simulink model "IFACS_Spring2026"  (R2025b)
settings: Solver=ode23t  StartTime=0.0  StopTime=3600*24*3  FixedStep=1  RelTol=1e-3  AbsTol=1e-3
values from neighbouring files (symbols this model uses):
  ac_cooling_capacity = 5000    [IFACS_Constants.m]
  ac_power = ac_cooling_capacity / ac_COP    (= 1250)    [IFACS_Constants.m]
  house_H = 6    [IFACS_Constants.m]
  house_L = 20    [IFACS_Constants.m]
  house_W = 10    [IFACS_Constants.m]
  roof_pitch = 15    [IFACS_Constants.m]
  TinIC = 24    [IFACS_Constants.m]
libraries: fl_lib x215, nesl_utility x52, simulink_extras x29, SimscapeFluids_lib x3
(part 4 of 5)

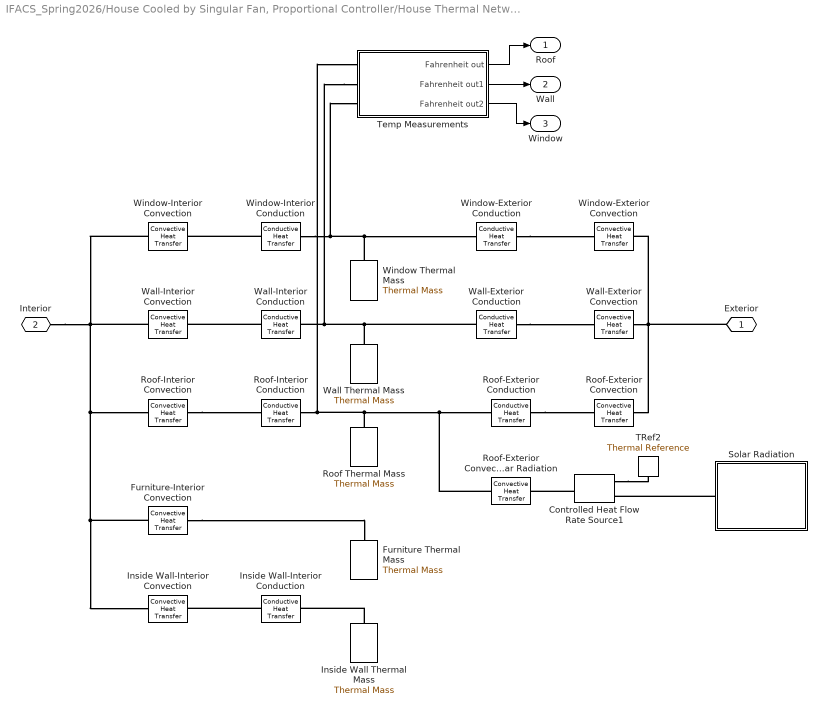
== system IFACS_Spring2026/House Cooled by Singular Fan, Proportional Controller/House Thermal Network/House Thermal Network ==
  Controlled Heat Flow Rate Source1 : fl_lib/Thermal/Thermal Sources/Controlled Heat Flow Rate Source
  Furniture Thermal Mass : fl_lib/Thermal/Thermal Elements/Thermal Mass  mass_type=foundation.enum.constant_variable.constant  mass=M_furniture kg  sp_heat=cp_furniture J/(K*kg)  mass_min=1e-6 kg  num_ports=foundation.enum.numPorts2.one  m_specify=off  m_priority=High  m=1 kg  m_nominal_specify=off  m_nominal_value=1  m_nominal_unit=kg  T_specify=on  T_priority=High  T=T_init_furniture degC  T_nominal_specify=off  T_nominal_value=1  T_nominal_unit=K  Q_specify=off  Q_priority=None  Q=0 W  Q_nominal_specify=off  Q_nominal_value=1  Q_nominal_unit=W
  Furniture-Interior Convection : fl_lib/Thermal/Thermal Elements/Convective Heat Transfer  thermal_type=foundation.enum.constant_variable.constant  area=area_furniture m^2  heat_tr_coeff=hc_furniture_interior W/(K*m^2)  min_heat_tr_coeff=1e-3 W/(K*m^2)  T_specify=off  T_priority=None  T=0 K  T_nominal_specify=off  T_nominal_value=1  T_nominal_unit=K  Q_specify=off  Q_priority=None  Q=0 W  Q_nominal_specify=off  Q_nominal_value=1  Q_nominal_unit=W
  Inside Wall Thermal Mass : fl_lib/Thermal/Thermal Elements/Thermal Mass  mass_type=foundation.enum.constant_variable.constant  mass=rho_wall_inside * area_wall_inside * thickness_wall_inside kg  sp_heat=cp_wall_inside J/(K*kg)  mass_min=1e-6 kg  num_ports=foundation.enum.numPorts2.one  m_specify=off  m_priority=High  m=1 kg  m_nominal_specify=off  m_nominal_value=1  m_nominal_unit=kg  T_specify=on  T_priority=High  T=T_init_wall_inside degC  T_nominal_specify=off  T_nominal_value=1  T_nominal_unit=K  Q_specify=off  Q_priority=None  Q=0 W  Q_nominal_specify=off  Q_nominal_value=1  Q_nominal_unit=W
  Inside Wall-Interior Conduction : fl_lib/Thermal/Thermal Elements/Conductive Heat Transfer  thermal_type=foundation.enum.ConstantVariableTabulated.Constant  wall_geometry=foundation.enum.ConductionWallGeometry.Planar  area=2 * area_wall_inside m^2  thickness=thickness_wall_inside / 2 m  d_in=0.05 m  d_out=0.1 m  L=1 m  th_cond_min=10 W/(K*m)  th_cond=k_wall_inside W/(K*m)  th_cond_TLU=[413, 401, 392, 383, 371, 357, 342] W/(K*m)  temp_TLU=[200, 273, 400, 600, 800, 1000, 1200] K  T_specify=off  T_priority=None  T=0 K  T_nominal_specify=off  T_nominal_value=1  T_nominal_unit=K  Q_specify=off  Q_priority=None  Q=0 W  Q_nominal_specify=off  Q_nominal_value=1  Q_nominal_unit=W
  Inside Wall-Interior Convection : fl_lib/Thermal/Thermal Elements/Convective Heat Transfer  thermal_type=foundation.enum.constant_variable.constant  area=2 * area_wall_inside m^2  heat_tr_coeff=hc_wall_inside_interior W/(K*m^2)  min_heat_tr_coeff=1e-3 W/(K*m^2)  T_specify=off  T_priority=None  T=0 K  T_nominal_specify=off  T_nominal_value=1  T_nominal_unit=K  Q_specify=off  Q_priority=None  Q=0 W  Q_nominal_specify=off  Q_nominal_value=1  Q_nominal_unit=W
  Roof Thermal Mass : fl_lib/Thermal/Thermal Elements/Thermal Mass  mass_type=foundation.enum.constant_variable.constant  mass=rho_roof * area_roof * thickness_roof kg  sp_heat=cp_roof J/(K*kg)  mass_min=1e-6 kg  num_ports=foundation.enum.numPorts2.one  m_specify=off  m_priority=High  m=1 kg  m_nominal_specify=off  m_nominal_value=1  m_nominal_unit=kg  T_specify=on  T_priority=High  T=T_init_roof degC  T_nominal_specify=off  T_nominal_value=1  T_nominal_unit=K  Q_specify=off  Q_priority=None  Q=0 W  Q_nominal_specify=off  Q_nominal_value=1  Q_nominal_unit=W
  Roof-Exterior Conduction : fl_lib/Thermal/Thermal Elements/Conductive Heat Transfer  thermal_type=foundation.enum.ConstantVariableTabulated.Constant  wall_geometry=foundation.enum.ConductionWallGeometry.Planar  area=area_roof m^2  thickness=thickness_roof / 2 m  d_in=0.05 m  d_out=0.1 m  L=1 m  th_cond_min=10 W/(K*m)  th_cond=k_roof W/(K*m)  th_cond_TLU=[413, 401, 392, 383, 371, 357, 342] W/(K*m)  temp_TLU=[200, 273, 400, 600, 800, 1000, 1200] K  T_specify=off  T_priority=None  T=0 K  T_nominal_specify=off  T_nominal_value=1  T_nominal_unit=K  Q_specify=off  Q_priority=None  Q=0 W  Q_nominal_specify=off  Q_nominal_value=1  Q_nominal_unit=W
  Roof-Exterior Convection : fl_lib/Thermal/Thermal Elements/Convective Heat Transfer  thermal_type=foundation.enum.constant_variable.constant  area=area_roof m^2  heat_tr_coeff=hc_roof_exterior W/(K*m^2)  min_heat_tr_coeff=1e-3 W/(K*m^2)  T_specify=off  T_priority=None  T=0 K  T_nominal_specify=off  T_nominal_value=1  T_nominal_unit=K  Q_specify=off  Q_priority=None  Q=0 W  Q_nominal_specify=off  Q_nominal_value=1  Q_nominal_unit=W
  Roof-Exterior Convection Solar Radiation : fl_lib/Thermal/Thermal Elements/Convective Heat Transfer  thermal_type=foundation.enum.constant_variable.constant  area=area_roof m^2  heat_tr_coeff=1 W/(K*m^2)  min_heat_tr_coeff=1e-3 W/(K*m^2)  T_specify=off  T_priority=None  T=0 K  T_nominal_specify=off  T_nominal_value=1  T_nominal_unit=K  Q_specify=off  Q_priority=None  Q=0 W  Q_nominal_specify=off  Q_nominal_value=1  Q_nominal_unit=W
  Roof-Interior Conduction : fl_lib/Thermal/Thermal Elements/Conductive Heat Transfer  thermal_type=foundation.enum.ConstantVariableTabulated.Constant  wall_geometry=foundation.enum.ConductionWallGeometry.Planar  area=area_roof m^2  thickness=thickness_roof / 2 m  d_in=0.05 m  d_out=0.1 m  L=1 m  th_cond_min=10 W/(K*m)  th_cond=k_roof W/(K*m)  th_cond_TLU=[413, 401, 392, 383, 371, 357, 342] W/(K*m)  temp_TLU=[200, 273, 400, 600, 800, 1000, 1200] K  T_specify=off  T_priority=None  T=0 K  T_nominal_specify=off  T_nominal_value=1  T_nominal_unit=K  Q_specify=off  Q_priority=None  Q=0 W  Q_nominal_specify=off  Q_nominal_value=1  Q_nominal_unit=W
  Roof-Interior Convection : fl_lib/Thermal/Thermal Elements/Convective Heat Transfer  thermal_type=foundation.enum.constant_variable.constant  area=area_roof m^2  heat_tr_coeff=hc_roof_interior W/(K*m^2)  min_heat_tr_coeff=1e-3 W/(K*m^2)  T_specify=off  T_priority=None  T=0 K  T_nominal_specify=off  T_nominal_value=1  T_nominal_unit=K  Q_specify=off  Q_priority=None  Q=0 W  Q_nominal_specify=off  Q_nominal_value=1  Q_nominal_unit=W
  Solar Radiation : Subsystem
  TRef2 : fl_lib/Thermal/Thermal Elements/Thermal Reference
  Temp Measurements : Subsystem
  Wall Thermal Mass : fl_lib/Thermal/Thermal Elements/Thermal Mass  mass_type=foundation.enum.constant_variable.constant  mass=rho_wall * area_wall * thickness_wall kg  sp_heat=cp_wall J/(K*kg)  mass_min=1e-6 kg  num_ports=foundation.enum.numPorts2.one  m_specify=off  m_priority=High  m=1 kg  m_nominal_specify=off  m_nominal_value=1  m_nominal_unit=kg  T_specify=on  T_priority=High  T=T_init_wall degC  T_nominal_specify=off  T_nominal_value=1  T_nominal_unit=K  Q_specify=off  Q_priority=None  Q=0 W  Q_nominal_specify=off  Q_nominal_value=1  Q_nominal_unit=W
  Wall-Exterior Conduction : fl_lib/Thermal/Thermal Elements/Conductive Heat Transfer  thermal_type=foundation.enum.ConstantVariableTabulated.Constant  wall_geometry=foundation.enum.ConductionWallGeometry.Planar  area=area_wall m^2  thickness=thickness_wall / 2 m  d_in=0.05 m  d_out=0.1 m  L=1 m  th_cond_min=10 W/(K*m)  th_cond=k_wall W/(K*m)  th_cond_TLU=[413, 401, 392, 383, 371, 357, 342] W/(K*m)  temp_TLU=[200, 273, 400, 600, 800, 1000, 1200] K  T_specify=off  T_priority=None  T=0 K  T_nominal_specify=off  T_nominal_value=1  T_nominal_unit=K  Q_specify=off  Q_priority=None  Q=0 W  Q_nominal_specify=off  Q_nominal_value=1  Q_nominal_unit=W
  Wall-Exterior Convection : fl_lib/Thermal/Thermal Elements/Convective Heat Transfer  thermal_type=foundation.enum.constant_variable.constant  area=area_wall m^2  heat_tr_coeff=hc_wall_exterior W/(K*m^2)  min_heat_tr_coeff=1e-3 W/(K*m^2)  T_specify=off  T_priority=None  T=0 K  T_nominal_specify=off  T_nominal_value=1  T_nominal_unit=K  Q_specify=off  Q_priority=None  Q=0 W  Q_nominal_specify=off  Q_nominal_value=1  Q_nominal_unit=W
  Wall-Interior Conduction : fl_lib/Thermal/Thermal Elements/Conductive Heat Transfer  thermal_type=foundation.enum.ConstantVariableTabulated.Constant  wall_geometry=foundation.enum.ConductionWallGeometry.Planar  area=area_wall m^2  thickness=thickness_wall / 2 m  d_in=0.05 m  d_out=0.1 m  L=1 m  th_cond_min=10 W/(K*m)  th_cond=k_wall W/(K*m)  th_cond_TLU=[413, 401, 392, 383, 371, 357, 342] W/(K*m)  temp_TLU=[200, 273, 400, 600, 800, 1000, 1200] K  T_specify=off  T_priority=None  T=0 K  T_nominal_specify=off  T_nominal_value=1  T_nominal_unit=K  Q_specify=off  Q_priority=None  Q=0 W  Q_nominal_specify=off  Q_nominal_value=1  Q_nominal_unit=W
  Wall-Interior Convection : fl_lib/Thermal/Thermal Elements/Convective Heat Transfer  thermal_type=foundation.enum.constant_variable.constant  area=area_wall m^2  heat_tr_coeff=hc_wall_interior W/(K*m^2)  min_heat_tr_coeff=1e-3 W/(K*m^2)  T_specify=off  T_priority=None  T=0 K  T_nominal_specify=off  T_nominal_value=1  T_nominal_unit=K  Q_specify=off  Q_priority=None  Q=0 W  Q_nominal_specify=off  Q_nominal_value=1  Q_nominal_unit=W
  Window Thermal Mass : fl_lib/Thermal/Thermal Elements/Thermal Mass  mass_type=foundation.enum.constant_variable.constant  mass=rho_window * area_window * thickness_window kg  sp_heat=cp_window J/(K*kg)  mass_min=1e-6 kg  num_ports=foundation.enum.numPorts2.one  m_specify=off  m_priority=High  m=1 kg  m_nominal_specify=off  m_nominal_value=1  m_nominal_unit=kg  T_specify=on  T_priority=High  T=T_init_window degC  T_nominal_specify=off  T_nominal_value=1  T_nominal_unit=K  Q_specify=off  Q_priority=None  Q=0 W  Q_nominal_specify=off  Q_nominal_value=1  Q_nominal_unit=W
  Window-Exterior Conduction : fl_lib/Thermal/Thermal Elements/Conductive Heat Transfer  thermal_type=foundation.enum.ConstantVariableTabulated.Constant  wall_geometry=foundation.enum.ConductionWallGeometry.Planar  area=area_window m^2  thickness=thickness_window / 2 m  d_in=0.05 m  d_out=0.1 m  L=1 m  th_cond_min=10 W/(K*m)  th_cond=k_window W/(K*m)  th_cond_TLU=[413, 401, 392, 383, 371, 357, 342] W/(K*m)  temp_TLU=[200, 273, 400, 600, 800, 1000, 1200] K  T_specify=off  T_priority=None  T=0 K  T_nominal_specify=off  T_nominal_value=1  T_nominal_unit=K  Q_specify=off  Q_priority=None  Q=0 W  Q_nominal_specify=off  Q_nominal_value=1  Q_nominal_unit=W
  Window-Exterior Convection : fl_lib/Thermal/Thermal Elements/Convective Heat Transfer  thermal_type=foundation.enum.constant_variable.constant  area=area_window m^2  heat_tr_coeff=hc_window_exterior W/(K*m^2)  min_heat_tr_coeff=1e-3 W/(K*m^2)  T_specify=off  T_priority=None  T=0 K  T_nominal_specify=off  T_nominal_value=1  T_nominal_unit=K  Q_specify=off  Q_priority=None  Q=0 W  Q_nominal_specify=off  Q_nominal_value=1  Q_nominal_unit=W
  Window-Interior Conduction : fl_lib/Thermal/Thermal Elements/Conductive Heat Transfer  thermal_type=foundation.enum.ConstantVariableTabulated.Constant  wall_geometry=foundation.enum.ConductionWallGeometry.Planar  area=area_window m^2  thickness=thickness_window / 2 m  d_in=0.05 m  d_out=0.1 m  L=1 m  th_cond_min=10 W/(K*m)  th_cond=k_window W/(K*m)  th_cond_TLU=[413, 401, 392, 383, 371, 357, 342] W/(K*m)  temp_TLU=[200, 273, 400, 600, 800, 1000, 1200] K  T_specify=off  T_priority=None  T=0 K  T_nominal_specify=off  T_nominal_value=1  T_nominal_unit=K  Q_specify=off  Q_priority=None  Q=0 W  Q_nominal_specify=off  Q_nominal_value=1  Q_nominal_unit=W
  Window-Interior Convection : fl_lib/Thermal/Thermal Elements/Convective Heat Transfer  thermal_type=foundation.enum.constant_variable.constant  area=area_window m^2  heat_tr_coeff=hc_window_interior W/(K*m^2)  min_heat_tr_coeff=1e-3 W/(K*m^2)  T_specify=off  T_priority=None  T=0 K  T_nominal_specify=off  T_nominal_value=1  T_nominal_unit=K  Q_specify=off  Q_priority=None  Q=0 W  Q_nominal_specify=off  Q_nominal_value=1  Q_nominal_unit=W
  Exterior : PMIOPort  Side=Left
  Interior : PMIOPort  Port=2  Side=Right
  Roof : Outport  VectorParamsAs1DForOutWhenUnconnected=off
  Wall : Outport  Port=2  VectorParamsAs1DForOutWhenUnconnected=off
  Window : Outport  Port=3  VectorParamsAs1DForOutWhenUnconnected=off
  wires:
  Temp Measurements/1(Fahrenheit out) -> Roof/1
  Temp Measurements/3(Fahrenheit out2) -> Window/1
  Temp Measurements/2(Fahrenheit out1) -> Wall/1
  connections:
  Roof-Interior Convection/LConn1 -- Roof-Interior Conduction/RConn1
  Roof Thermal Mass/LConn1 -- Roof-Interior Conduction/LConn1 -- Temp Measurements/LConn1 -- Roof-Exterior Convection Solar Radiation/RConn1 -- Roof-Exterior Conduction/RConn1
  Roof-Exterior Conduction/LConn1 -- Roof-Exterior Convection/RConn1
  Temp Measurements/LConn2 -- Wall-Interior Conduction/LConn1 -- Wall Thermal Mass/LConn1 -- Wall-Exterior Conduction/RConn1
  Wall-Interior Conduction/RConn1 -- Wall-Interior Convection/LConn1
  Wall-Exterior Conduction/LConn1 -- Wall-Exterior Convection/RConn1
  Window-Interior Conduction/RConn1 -- Window-Interior Convection/LConn1
  Window-Interior Conduction/LConn1 -- Temp Measurements/LConn3 -- Window Thermal Mass/LConn1 -- Window-Exterior Conduction/RConn1
  Window-Exterior Conduction/LConn1 -- Window-Exterior Convection/RConn1
  Inside Wall Thermal Mass/LConn1 -- Inside Wall-Interior Conduction/LConn1
  Furniture-Interior Convection/RConn1 -- Window-Interior Convection/RConn1 -- Wall-Interior Convection/RConn1 -- Interior/RConn1 -- Roof-Interior Convection/RConn1 -- Inside Wall-Interior Convection/RConn1
  Inside Wall-Interior Conduction/RConn1 -- Inside Wall-Interior Convection/LConn1
  Furniture-Interior Convection/LConn1 -- Furniture Thermal Mass/LConn1
  Roof-Exterior Convection/LConn1 -- Exterior/RConn1 -- Window-Exterior Convection/LConn1 -- Wall-Exterior Convection/LConn1
  Controlled Heat Flow Rate Source1/RConn2 -- TRef2/LConn1
  Controlled Heat Flow Rate Source1/LConn1 -- Roof-Exterior Convection Solar Radiation/LConn1
  Solar Radiation/RConn1 -- Controlled Heat Flow Rate Source1/RConn1

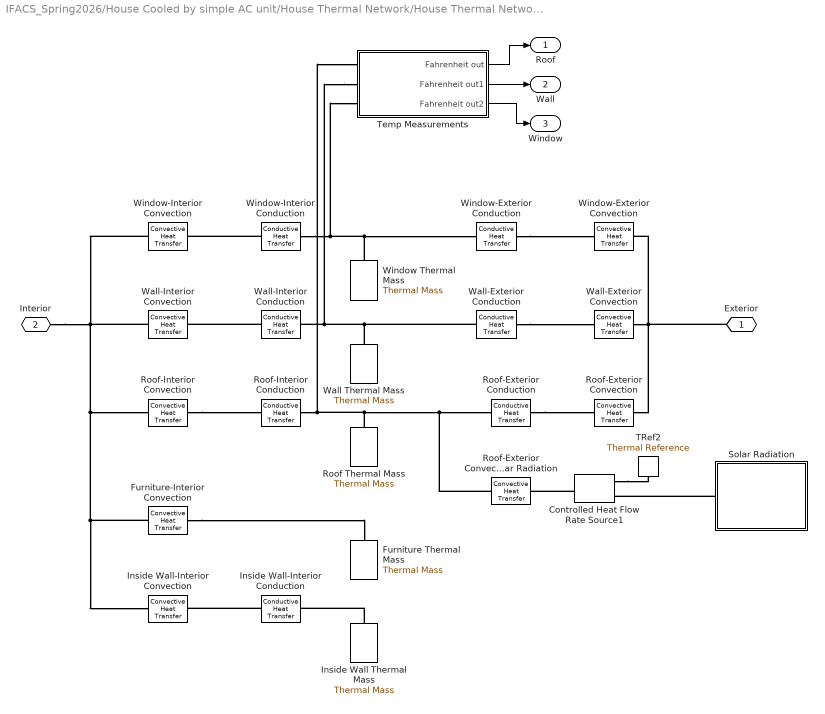
== system IFACS_Spring2026/House Cooled by simple AC unit/House Thermal Network/House Thermal Network ==
  Controlled Heat Flow Rate Source1 : fl_lib/Thermal/Thermal Sources/Controlled Heat Flow Rate Source
  Furniture Thermal Mass : fl_lib/Thermal/Thermal Elements/Thermal Mass  mass_type=foundation.enum.constant_variable.constant  mass=M_furniture kg  sp_heat=cp_furniture J/(K*kg)  mass_min=1e-6 kg  num_ports=foundation.enum.numPorts2.one  m_specify=off  m_priority=High  m=1 kg  m_nominal_specify=off  m_nominal_value=1  m_nominal_unit=kg  T_specify=on  T_priority=High  T=T_init_furniture degC  T_nominal_specify=off  T_nominal_value=1  T_nominal_unit=K  Q_specify=off  Q_priority=None  Q=0 W  Q_nominal_specify=off  Q_nominal_value=1  Q_nominal_unit=W
  Furniture-Interior Convection : fl_lib/Thermal/Thermal Elements/Convective Heat Transfer  thermal_type=foundation.enum.constant_variable.constant  area=area_furniture m^2  heat_tr_coeff=hc_furniture_interior W/(K*m^2)  min_heat_tr_coeff=1e-3 W/(K*m^2)  T_specify=off  T_priority=None  T=0 K  T_nominal_specify=off  T_nominal_value=1  T_nominal_unit=K  Q_specify=off  Q_priority=None  Q=0 W  Q_nominal_specify=off  Q_nominal_value=1  Q_nominal_unit=W
  Inside Wall Thermal Mass : fl_lib/Thermal/Thermal Elements/Thermal Mass  mass_type=foundation.enum.constant_variable.constant  mass=rho_wall_inside * area_wall_inside * thickness_wall_inside kg  sp_heat=cp_wall_inside J/(K*kg)  mass_min=1e-6 kg  num_ports=foundation.enum.numPorts2.one  m_specify=off  m_priority=High  m=1 kg  m_nominal_specify=off  m_nominal_value=1  m_nominal_unit=kg  T_specify=on  T_priority=High  T=T_init_wall_inside degC  T_nominal_specify=off  T_nominal_value=1  T_nominal_unit=K  Q_specify=off  Q_priority=None  Q=0 W  Q_nominal_specify=off  Q_nominal_value=1  Q_nominal_unit=W
  Inside Wall-Interior Conduction : fl_lib/Thermal/Thermal Elements/Conductive Heat Transfer  thermal_type=foundation.enum.ConstantVariableTabulated.Constant  wall_geometry=foundation.enum.ConductionWallGeometry.Planar  area=2 * area_wall_inside m^2  thickness=thickness_wall_inside / 2 m  d_in=0.05 m  d_out=0.1 m  L=1 m  th_cond_min=10 W/(K*m)  th_cond=k_wall_inside W/(K*m)  th_cond_TLU=[413, 401, 392, 383, 371, 357, 342] W/(K*m)  temp_TLU=[200, 273, 400, 600, 800, 1000, 1200] K  T_specify=off  T_priority=None  T=0 K  T_nominal_specify=off  T_nominal_value=1  T_nominal_unit=K  Q_specify=off  Q_priority=None  Q=0 W  Q_nominal_specify=off  Q_nominal_value=1  Q_nominal_unit=W
  Inside Wall-Interior Convection : fl_lib/Thermal/Thermal Elements/Convective Heat Transfer  thermal_type=foundation.enum.constant_variable.constant  area=2 * area_wall_inside m^2  heat_tr_coeff=hc_wall_inside_interior W/(K*m^2)  min_heat_tr_coeff=1e-3 W/(K*m^2)  T_specify=off  T_priority=None  T=0 K  T_nominal_specify=off  T_nominal_value=1  T_nominal_unit=K  Q_specify=off  Q_priority=None  Q=0 W  Q_nominal_specify=off  Q_nominal_value=1  Q_nominal_unit=W
  Roof Thermal Mass : fl_lib/Thermal/Thermal Elements/Thermal Mass  mass_type=foundation.enum.constant_variable.constant  mass=rho_roof * area_roof * thickness_roof kg  sp_heat=cp_roof J/(K*kg)  mass_min=1e-6 kg  num_ports=foundation.enum.numPorts2.one  m_specify=off  m_priority=High  m=1 kg  m_nominal_specify=off  m_nominal_value=1  m_nominal_unit=kg  T_specify=on  T_priority=High  T=T_init_roof degC  T_nominal_specify=off  T_nominal_value=1  T_nominal_unit=K  Q_specify=off  Q_priority=None  Q=0 W  Q_nominal_specify=off  Q_nominal_value=1  Q_nominal_unit=W
  Roof-Exterior Conduction : fl_lib/Thermal/Thermal Elements/Conductive Heat Transfer  thermal_type=foundation.enum.ConstantVariableTabulated.Constant  wall_geometry=foundation.enum.ConductionWallGeometry.Planar  area=area_roof m^2  thickness=thickness_roof / 2 m  d_in=0.05 m  d_out=0.1 m  L=1 m  th_cond_min=10 W/(K*m)  th_cond=k_roof W/(K*m)  th_cond_TLU=[413, 401, 392, 383, 371, 357, 342] W/(K*m)  temp_TLU=[200, 273, 400, 600, 800, 1000, 1200] K  T_specify=off  T_priority=None  T=0 K  T_nominal_specify=off  T_nominal_value=1  T_nominal_unit=K  Q_specify=off  Q_priority=None  Q=0 W  Q_nominal_specify=off  Q_nominal_value=1  Q_nominal_unit=W
  Roof-Exterior Convection : fl_lib/Thermal/Thermal Elements/Convective Heat Transfer  thermal_type=foundation.enum.constant_variable.constant  area=area_roof m^2  heat_tr_coeff=hc_roof_exterior W/(K*m^2)  min_heat_tr_coeff=1e-3 W/(K*m^2)  T_specify=off  T_priority=None  T=0 K  T_nominal_specify=off  T_nominal_value=1  T_nominal_unit=K  Q_specify=off  Q_priority=None  Q=0 W  Q_nominal_specify=off  Q_nominal_value=1  Q_nominal_unit=W
  Roof-Exterior Convection Solar Radiation : fl_lib/Thermal/Thermal Elements/Convective Heat Transfer  thermal_type=foundation.enum.constant_variable.constant  area=area_roof m^2  heat_tr_coeff=1 W/(K*m^2)  min_heat_tr_coeff=1e-3 W/(K*m^2)  T_specify=off  T_priority=None  T=0 K  T_nominal_specify=off  T_nominal_value=1  T_nominal_unit=K  Q_specify=off  Q_priority=None  Q=0 W  Q_nominal_specify=off  Q_nominal_value=1  Q_nominal_unit=W
  Roof-Interior Conduction : fl_lib/Thermal/Thermal Elements/Conductive Heat Transfer  thermal_type=foundation.enum.ConstantVariableTabulated.Constant  wall_geometry=foundation.enum.ConductionWallGeometry.Planar  area=area_roof m^2  thickness=thickness_roof / 2 m  d_in=0.05 m  d_out=0.1 m  L=1 m  th_cond_min=10 W/(K*m)  th_cond=k_roof W/(K*m)  th_cond_TLU=[413, 401, 392, 383, 371, 357, 342] W/(K*m)  temp_TLU=[200, 273, 400, 600, 800, 1000, 1200] K  T_specify=off  T_priority=None  T=0 K  T_nominal_specify=off  T_nominal_value=1  T_nominal_unit=K  Q_specify=off  Q_priority=None  Q=0 W  Q_nominal_specify=off  Q_nominal_value=1  Q_nominal_unit=W
  Roof-Interior Convection : fl_lib/Thermal/Thermal Elements/Convective Heat Transfer  thermal_type=foundation.enum.constant_variable.constant  area=area_roof m^2  heat_tr_coeff=hc_roof_interior W/(K*m^2)  min_heat_tr_coeff=1e-3 W/(K*m^2)  T_specify=off  T_priority=None  T=0 K  T_nominal_specify=off  T_nominal_value=1  T_nominal_unit=K  Q_specify=off  Q_priority=None  Q=0 W  Q_nominal_specify=off  Q_nominal_value=1  Q_nominal_unit=W
  Solar Radiation : Subsystem
  TRef2 : fl_lib/Thermal/Thermal Elements/Thermal Reference
  Temp Measurements : Subsystem
  Wall Thermal Mass : fl_lib/Thermal/Thermal Elements/Thermal Mass  mass_type=foundation.enum.constant_variable.constant  mass=rho_wall * area_wall * thickness_wall kg  sp_heat=cp_wall J/(K*kg)  mass_min=1e-6 kg  num_ports=foundation.enum.numPorts2.one  m_specify=off  m_priority=High  m=1 kg  m_nominal_specify=off  m_nominal_value=1  m_nominal_unit=kg  T_specify=on  T_priority=High  T=T_init_wall degC  T_nominal_specify=off  T_nominal_value=1  T_nominal_unit=K  Q_specify=off  Q_priority=None  Q=0 W  Q_nominal_specify=off  Q_nominal_value=1  Q_nominal_unit=W
  Wall-Exterior Conduction : fl_lib/Thermal/Thermal Elements/Conductive Heat Transfer  thermal_type=foundation.enum.ConstantVariableTabulated.Constant  wall_geometry=foundation.enum.ConductionWallGeometry.Planar  area=area_wall m^2  thickness=thickness_wall / 2 m  d_in=0.05 m  d_out=0.1 m  L=1 m  th_cond_min=10 W/(K*m)  th_cond=k_wall W/(K*m)  th_cond_TLU=[413, 401, 392, 383, 371, 357, 342] W/(K*m)  temp_TLU=[200, 273, 400, 600, 800, 1000, 1200] K  T_specify=off  T_priority=None  T=0 K  T_nominal_specify=off  T_nominal_value=1  T_nominal_unit=K  Q_specify=off  Q_priority=None  Q=0 W  Q_nominal_specify=off  Q_nominal_value=1  Q_nominal_unit=W
  Wall-Exterior Convection : fl_lib/Thermal/Thermal Elements/Convective Heat Transfer  thermal_type=foundation.enum.constant_variable.constant  area=area_wall m^2  heat_tr_coeff=hc_wall_exterior W/(K*m^2)  min_heat_tr_coeff=1e-3 W/(K*m^2)  T_specify=off  T_priority=None  T=0 K  T_nominal_specify=off  T_nominal_value=1  T_nominal_unit=K  Q_specify=off  Q_priority=None  Q=0 W  Q_nominal_specify=off  Q_nominal_value=1  Q_nominal_unit=W
  Wall-Interior Conduction : fl_lib/Thermal/Thermal Elements/Conductive Heat Transfer  thermal_type=foundation.enum.ConstantVariableTabulated.Constant  wall_geometry=foundation.enum.ConductionWallGeometry.Planar  area=area_wall m^2  thickness=thickness_wall / 2 m  d_in=0.05 m  d_out=0.1 m  L=1 m  th_cond_min=10 W/(K*m)  th_cond=k_wall W/(K*m)  th_cond_TLU=[413, 401, 392, 383, 371, 357, 342] W/(K*m)  temp_TLU=[200, 273, 400, 600, 800, 1000, 1200] K  T_specify=off  T_priority=None  T=0 K  T_nominal_specify=off  T_nominal_value=1  T_nominal_unit=K  Q_specify=off  Q_priority=None  Q=0 W  Q_nominal_specify=off  Q_nominal_value=1  Q_nominal_unit=W
  Wall-Interior Convection : fl_lib/Thermal/Thermal Elements/Convective Heat Transfer  thermal_type=foundation.enum.constant_variable.constant  area=area_wall m^2  heat_tr_coeff=hc_wall_interior W/(K*m^2)  min_heat_tr_coeff=1e-3 W/(K*m^2)  T_specify=off  T_priority=None  T=0 K  T_nominal_specify=off  T_nominal_value=1  T_nominal_unit=K  Q_specify=off  Q_priority=None  Q=0 W  Q_nominal_specify=off  Q_nominal_value=1  Q_nominal_unit=W
  Window Thermal Mass : fl_lib/Thermal/Thermal Elements/Thermal Mass  mass_type=foundation.enum.constant_variable.constant  mass=rho_window * area_window * thickness_window kg  sp_heat=cp_window J/(K*kg)  mass_min=1e-6 kg  num_ports=foundation.enum.numPorts2.one  m_specify=off  m_priority=High  m=1 kg  m_nominal_specify=off  m_nominal_value=1  m_nominal_unit=kg  T_specify=on  T_priority=High  T=T_init_window degC  T_nominal_specify=off  T_nominal_value=1  T_nominal_unit=K  Q_specify=off  Q_priority=None  Q=0 W  Q_nominal_specify=off  Q_nominal_value=1  Q_nominal_unit=W
  Window-Exterior Conduction : fl_lib/Thermal/Thermal Elements/Conductive Heat Transfer  thermal_type=foundation.enum.ConstantVariableTabulated.Constant  wall_geometry=foundation.enum.ConductionWallGeometry.Planar  area=area_window m^2  thickness=thickness_window / 2 m  d_in=0.05 m  d_out=0.1 m  L=1 m  th_cond_min=10 W/(K*m)  th_cond=k_window W/(K*m)  th_cond_TLU=[413, 401, 392, 383, 371, 357, 342] W/(K*m)  temp_TLU=[200, 273, 400, 600, 800, 1000, 1200] K  T_specify=off  T_priority=None  T=0 K  T_nominal_specify=off  T_nominal_value=1  T_nominal_unit=K  Q_specify=off  Q_priority=None  Q=0 W  Q_nominal_specify=off  Q_nominal_value=1  Q_nominal_unit=W
  Window-Exterior Convection : fl_lib/Thermal/Thermal Elements/Convective Heat Transfer  thermal_type=foundation.enum.constant_variable.constant  area=area_window m^2  heat_tr_coeff=hc_window_exterior W/(K*m^2)  min_heat_tr_coeff=1e-3 W/(K*m^2)  T_specify=off  T_priority=None  T=0 K  T_nominal_specify=off  T_nominal_value=1  T_nominal_unit=K  Q_specify=off  Q_priority=None  Q=0 W  Q_nominal_specify=off  Q_nominal_value=1  Q_nominal_unit=W
  Window-Interior Conduction : fl_lib/Thermal/Thermal Elements/Conductive Heat Transfer  thermal_type=foundation.enum.ConstantVariableTabulated.Constant  wall_geometry=foundation.enum.ConductionWallGeometry.Planar  area=area_window m^2  thickness=thickness_window / 2 m  d_in=0.05 m  d_out=0.1 m  L=1 m  th_cond_min=10 W/(K*m)  th_cond=k_window W/(K*m)  th_cond_TLU=[413, 401, 392, 383, 371, 357, 342] W/(K*m)  temp_TLU=[200, 273, 400, 600, 800, 1000, 1200] K  T_specify=off  T_priority=None  T=0 K  T_nominal_specify=off  T_nominal_value=1  T_nominal_unit=K  Q_specify=off  Q_priority=None  Q=0 W  Q_nominal_specify=off  Q_nominal_value=1  Q_nominal_unit=W
  Window-Interior Convection : fl_lib/Thermal/Thermal Elements/Convective Heat Transfer  thermal_type=foundation.enum.constant_variable.constant  area=area_window m^2  heat_tr_coeff=hc_window_interior W/(K*m^2)  min_heat_tr_coeff=1e-3 W/(K*m^2)  T_specify=off  T_priority=None  T=0 K  T_nominal_specify=off  T_nominal_value=1  T_nominal_unit=K  Q_specify=off  Q_priority=None  Q=0 W  Q_nominal_specify=off  Q_nominal_value=1  Q_nominal_unit=W
  Exterior : PMIOPort  Side=Left
  Interior : PMIOPort  Port=2  Side=Right
  Roof : Outport  VectorParamsAs1DForOutWhenUnconnected=off
  Wall : Outport  Port=2  VectorParamsAs1DForOutWhenUnconnected=off
  Window : Outport  Port=3  VectorParamsAs1DForOutWhenUnconnected=off
  wires:
  Temp Measurements/1(Fahrenheit out) -> Roof/1
  Temp Measurements/3(Fahrenheit out2) -> Window/1
  Temp Measurements/2(Fahrenheit out1) -> Wall/1
  connections:
  Roof-Interior Convection/LConn1 -- Roof-Interior Conduction/RConn1
  Roof Thermal Mass/LConn1 -- Roof-Interior Conduction/LConn1 -- Temp Measurements/LConn1 -- Roof-Exterior Convection Solar Radiation/RConn1 -- Roof-Exterior Conduction/RConn1
  Roof-Exterior Conduction/LConn1 -- Roof-Exterior Convection/RConn1
  Temp Measurements/LConn2 -- Wall-Interior Conduction/LConn1 -- Wall Thermal Mass/LConn1 -- Wall-Exterior Conduction/RConn1
  Wall-Interior Conduction/RConn1 -- Wall-Interior Convection/LConn1
  Wall-Exterior Conduction/LConn1 -- Wall-Exterior Convection/RConn1
  Window-Interior Conduction/RConn1 -- Window-Interior Convection/LConn1
  Window-Interior Conduction/LConn1 -- Temp Measurements/LConn3 -- Window Thermal Mass/LConn1 -- Window-Exterior Conduction/RConn1
  Window-Exterior Conduction/LConn1 -- Window-Exterior Convection/RConn1
  Inside Wall Thermal Mass/LConn1 -- Inside Wall-Interior Conduction/LConn1
  Furniture-Interior Convection/RConn1 -- Window-Interior Convection/RConn1 -- Wall-Interior Convection/RConn1 -- Interior/RConn1 -- Roof-Interior Convection/RConn1 -- Inside Wall-Interior Convection/RConn1
  Inside Wall-Interior Conduction/RConn1 -- Inside Wall-Interior Convection/LConn1
  Furniture-Interior Convection/LConn1 -- Furniture Thermal Mass/LConn1
  Roof-Exterior Convection/LConn1 -- Exterior/RConn1 -- Window-Exterior Convection/LConn1 -- Wall-Exterior Convection/LConn1
  Controlled Heat Flow Rate Source1/RConn2 -- TRef2/LConn1
  Controlled Heat Flow Rate Source1/LConn1 -- Roof-Exterior Convection Solar Radiation/LConn1
  Solar Radiation/RConn1 -- Controlled Heat Flow Rate Source1/RConn1

== system IFACS_Spring2026/House Thermal Network /House Thermal Network/Solar Radiation ==
  From Workspace : FromWorkspace  VariableName=time_radiation
  Product : Product
  Relay : Relay  OnSwitchValue=1  OffSwitchValue=0
  Scope : Scope  NumInputPorts=2
      settings: TimeUnits=Metric (based on Time Span)  ActiveDisplayYMinimum=-624.999986167378  ActiveDisplayYMaximum=5624.9998755064025  DataLoggingVariableName=ScopeData2
  Simulink-PS Converter1 : nesl_utility/Simulink-PS Converter  PhysicalDomain=network_engine_domain  SubClassName=ps_input  LeftPortType=input  RightPortType=output  PseudoPeriodic=off  Frequencies=[]  NoiseDistribution=none  NoiseParameters=[]  Unit=1  AffineConversion=off  FilteringAndDerivatives=provide  SimscapeFilterOrder=1  InputFilterTimeConstant=0.001  UdotUserProvided=0
  Solar Cycle : Sin  Amplitude=5000  Frequency=(2*pi)/(24*3600)  SampleTime=0
  Solar Radiation : PMIOPort  Side=Right
  wires:
  Relay/1 -> Product/2
  Solar Cycle/1 -> Product/1, Relay/1
  Product/1 -> Scope/2
  From Workspace/1 -> Simulink-PS Converter1/1, Scope/1
  connections:
  Simulink-PS Converter1/RConn1 -- Solar Radiation/RConn1

== system IFACS_Spring2026/House Thermal Network /House Thermal Network/Temp Measurements ==
  Celsius to Fahrenheit : simulink_extras/Transformations/Celsius to Fahrenheit
  Celsius to Fahrenheit1 : simulink_extras/Transformations/Celsius to Fahrenheit
  Celsius to Fahrenheit2 : simulink_extras/Transformations/Celsius to Fahrenheit
  PS2S1 : nesl_utility/PS-Simulink Converter  PhysicalDomain=network_engine_domain  SubClassName=ps_output  LeftPortType=input  RightPortType=output  PseudoPeriodic=off  Frequencies=[]  VectorFormat=1-D array  Unit=degC  AffineConversion=on
  PS2S2 : nesl_utility/PS-Simulink Converter  PhysicalDomain=network_engine_domain  SubClassName=ps_output  LeftPortType=input  RightPortType=output  PseudoPeriodic=off  Frequencies=[]  VectorFormat=1-D array  Unit=degC  AffineConversion=on
  PS2S3 : nesl_utility/PS-Simulink Converter  PhysicalDomain=network_engine_domain  SubClassName=ps_output  LeftPortType=input  RightPortType=output  PseudoPeriodic=off  Frequencies=[]  VectorFormat=1-D array  Unit=degC  AffineConversion=on
  TRef2 : fl_lib/Thermal/Thermal Elements/Thermal Reference
  TRef3 : fl_lib/Thermal/Thermal Elements/Thermal Reference
  TRef4 : fl_lib/Thermal/Thermal Elements/Thermal Reference
  Temperature Sensor1 : fl_lib/Thermal/Thermal Sensors/Temperature Sensor  temperature_measure=foundation.enum.MeasurementReference.difference
  Temperature Sensor2 : fl_lib/Thermal/Thermal Sensors/Temperature Sensor  temperature_measure=foundation.enum.MeasurementReference.difference
  Temperature Sensor3 : fl_lib/Thermal/Thermal Sensors/Temperature Sensor  temperature_measure=foundation.enum.MeasurementReference.difference
  Roof Temp : PMIOPort  Side=Left
  Wall Temp : PMIOPort  Port=2  Side=Left
  Window Temp : PMIOPort  Port=3  Side=Left
  Fahrenheit out : Outport
  Fahrenheit out1 : Outport  Port=2
  Fahrenheit out2 : Outport  Port=3
  wires:
  PS2S3/1 -> Celsius to Fahrenheit2/1  "Window"
  PS2S1/1 -> Celsius to Fahrenheit/1  "Roof"
  PS2S2/1 -> Celsius to Fahrenheit1/1  "Wall"
  Celsius to Fahrenheit2/1 -> Fahrenheit out2/1
  Celsius to Fahrenheit1/1 -> Fahrenheit out1/1
  Celsius to Fahrenheit/1 -> Fahrenheit out/1
  connections:
  PS2S2/LConn1 -- Temperature Sensor2/RConn2
  PS2S3/LConn1 -- Temperature Sensor3/RConn2
  TRef2/LConn1 -- Temperature Sensor1/RConn1
  TRef3/LConn1 -- Temperature Sensor2/RConn1
  PS2S1/LConn1 -- Temperature Sensor1/RConn2
  Temperature Sensor2/LConn1 -- Wall Temp/RConn1
  TRef4/LConn1 -- Temperature Sensor3/RConn1
  Temperature Sensor3/LConn1 -- Window Temp/RConn1
  Temperature Sensor1/LConn1 -- Roof Temp/RConn1

== system IFACS_Spring2026/House Cooled by AC and Singular Fan, Proportional Controller/Fan Parameters/Fan Activation/Fan Activation Relays ==
  Tmin : Inport
  Tenv : Inport  Port=2
  Troom : Inport  Port=3
  Cooling Activation : Relay  OnSwitchValue=1  OffSwitchValue=-1
  Product : Product
  Room Temp Min off switch : Relay  OnSwitchValue=2  OffSwitchValue=-2
  Sum1 : Sum  Inputs=-+|  InputSameDT=on  SaturateOnIntegerOverflow=on  OutDataTypeStr=Inherit: Same as first input
  Sum2 : Sum  Inputs=-+|  InputSameDT=on  SaturateOnIntegerOverflow=on  OutDataTypeStr=Inherit: Same as first input
  Fan Activation : Outport
  wires:
  Cooling Activation/1 -> Product/2  "1 if Troom > Tenv else 0"
  Sum2/1 -> Cooling Activation/1  "Terr"
  Tenv/1 -> Sum2/1
  Room Temp Min off switch/1 -> Product/1  "1 if Troom > Tmin else 0"
  Tmin/1 -> Sum1/1
  Troom/1 -> Sum1/2, Sum2/2
  Sum1/1 -> Room Temp Min off switch/1  "Terr"
  Product/1 -> Fan Activation/1

== system IFACS_Spring2026/House Cooled by AC and Singular Fan, Proportional Controller/House Thermal Network/House Thermal Network/Solar Radiation ==
  From Workspace : FromWorkspace  VariableName=time_radiation
  Product : Product
  Relay : Relay  OnSwitchValue=1  OffSwitchValue=0
  Scope : Scope  NumInputPorts=2
      settings: TimeUnits=Metric (based on Time Span)  ActiveDisplayYMinimum=-624.999986167378  ActiveDisplayYMaximum=5624.9998755064025  DataLoggingVariableName=ScopeData2
  Simulink-PS Converter1 : nesl_utility/Simulink-PS Converter  PhysicalDomain=network_engine_domain  SubClassName=ps_input  LeftPortType=input  RightPortType=output  PseudoPeriodic=off  Frequencies=[]  NoiseDistribution=none  NoiseParameters=[]  Unit=1  AffineConversion=off  FilteringAndDerivatives=provide  SimscapeFilterOrder=1  InputFilterTimeConstant=0.001  UdotUserProvided=0
  Solar Cycle : Sin  Amplitude=5000  Frequency=(2*pi)/(24*3600)  SampleTime=0
  Solar Radiation : PMIOPort  Side=Right
  wires:
  Relay/1 -> Product/2
  Solar Cycle/1 -> Product/1, Relay/1
  Product/1 -> Scope/2
  From Workspace/1 -> Simulink-PS Converter1/1, Scope/1
  connections:
  Simulink-PS Converter1/RConn1 -- Solar Radiation/RConn1

== system IFACS_Spring2026/House Cooled by AC and Singular Fan, Proportional Controller/House Thermal Network/House Thermal Network/Temp Measurements ==
  Celsius to Fahrenheit : simulink_extras/Transformations/Celsius to Fahrenheit
  Celsius to Fahrenheit1 : simulink_extras/Transformations/Celsius to Fahrenheit
  Celsius to Fahrenheit2 : simulink_extras/Transformations/Celsius to Fahrenheit
  PS2S1 : nesl_utility/PS-Simulink Converter  PhysicalDomain=network_engine_domain  SubClassName=ps_output  LeftPortType=input  RightPortType=output  PseudoPeriodic=off  Frequencies=[]  VectorFormat=1-D array  Unit=degC  AffineConversion=on
  PS2S2 : nesl_utility/PS-Simulink Converter  PhysicalDomain=network_engine_domain  SubClassName=ps_output  LeftPortType=input  RightPortType=output  PseudoPeriodic=off  Frequencies=[]  VectorFormat=1-D array  Unit=degC  AffineConversion=on
  PS2S3 : nesl_utility/PS-Simulink Converter  PhysicalDomain=network_engine_domain  SubClassName=ps_output  LeftPortType=input  RightPortType=output  PseudoPeriodic=off  Frequencies=[]  VectorFormat=1-D array  Unit=degC  AffineConversion=on
  TRef2 : fl_lib/Thermal/Thermal Elements/Thermal Reference
  TRef3 : fl_lib/Thermal/Thermal Elements/Thermal Reference
  TRef4 : fl_lib/Thermal/Thermal Elements/Thermal Reference
  Temperature Sensor1 : fl_lib/Thermal/Thermal Sensors/Temperature Sensor  temperature_measure=foundation.enum.MeasurementReference.difference
  Temperature Sensor2 : fl_lib/Thermal/Thermal Sensors/Temperature Sensor  temperature_measure=foundation.enum.MeasurementReference.difference
  Temperature Sensor3 : fl_lib/Thermal/Thermal Sensors/Temperature Sensor  temperature_measure=foundation.enum.MeasurementReference.difference
  Roof Temp : PMIOPort  Side=Left
  Wall Temp : PMIOPort  Port=2  Side=Left
  Window Temp : PMIOPort  Port=3  Side=Left
  Fahrenheit out : Outport
  Fahrenheit out1 : Outport  Port=2
  Fahrenheit out2 : Outport  Port=3
  wires:
  PS2S3/1 -> Celsius to Fahrenheit2/1  "Window"
  PS2S1/1 -> Celsius to Fahrenheit/1  "Roof"
  PS2S2/1 -> Celsius to Fahrenheit1/1  "Wall"
  Celsius to Fahrenheit2/1 -> Fahrenheit out2/1
  Celsius to Fahrenheit1/1 -> Fahrenheit out1/1
  Celsius to Fahrenheit/1 -> Fahrenheit out/1
  connections:
  PS2S2/LConn1 -- Temperature Sensor2/RConn2
  PS2S3/LConn1 -- Temperature Sensor3/RConn2
  TRef2/LConn1 -- Temperature Sensor1/RConn1
  TRef3/LConn1 -- Temperature Sensor2/RConn1
  PS2S1/LConn1 -- Temperature Sensor1/RConn2
  Temperature Sensor2/LConn1 -- Wall Temp/RConn1
  TRef4/LConn1 -- Temperature Sensor3/RConn1
  Temperature Sensor3/LConn1 -- Window Temp/RConn1
  Temperature Sensor1/LConn1 -- Roof Temp/RConn1

== system IFACS_Spring2026/House Cooled by Singular Fan, Bang Bang Controller/Fan Parameters/Fan Activation/Fan Activation Relays ==
  Tmin : Inport
  Tenv : Inport  Port=2
  Troom : Inport  Port=3
  Cooling Activation : Relay  OnSwitchValue=.001  OffSwitchValue=-1
  Product : Product
  Room Temp Min off switch : Relay  OnSwitchValue=.001  OffSwitchValue=-.001
  Sum1 : Sum  Inputs=-+|  InputSameDT=on  SaturateOnIntegerOverflow=on  OutDataTypeStr=Inherit: Same as first input
  Sum2 : Sum  Inputs=-+|  InputSameDT=on  SaturateOnIntegerOverflow=on  OutDataTypeStr=Inherit: Same as first input
  Fan Activation : Outport
  wires:
  Cooling Activation/1 -> Product/2  "1 if Troom > Tenv else 0"
  Sum2/1 -> Cooling Activation/1  "Terr"
  Tenv/1 -> Sum2/1
  Room Temp Min off switch/1 -> Product/1  "1 if Troom > Tmin else 0"
  Tmin/1 -> Sum1/1
  Troom/1 -> Sum1/2, Sum2/2
  Sum1/1 -> Room Temp Min off switch/1  "Terr"
  Product/1 -> Fan Activation/1

== system IFACS_Spring2026/House Cooled by Singular Fan, Bang Bang Controller/House Thermal Network/House Thermal Network/Solar Radiation ==
  From Workspace : FromWorkspace  VariableName=time_radiation
  Product : Product
  Relay : Relay  OnSwitchValue=1  OffSwitchValue=0
  Scope : Scope  NumInputPorts=2
      settings: TimeUnits=Metric (based on Time Span)  ActiveDisplayYMinimum=-624.999986167378  ActiveDisplayYMaximum=5624.9998755064025  DataLoggingVariableName=ScopeData2
  Simulink-PS Converter1 : nesl_utility/Simulink-PS Converter  PhysicalDomain=network_engine_domain  SubClassName=ps_input  LeftPortType=input  RightPortType=output  PseudoPeriodic=off  Frequencies=[]  NoiseDistribution=none  NoiseParameters=[]  Unit=1  AffineConversion=off  FilteringAndDerivatives=provide  SimscapeFilterOrder=1  InputFilterTimeConstant=0.001  UdotUserProvided=0
  Solar Cycle : Sin  Amplitude=5000  Frequency=(2*pi)/(24*3600)  SampleTime=0
  Solar Radiation : PMIOPort  Side=Right
  wires:
  Relay/1 -> Product/2
  Solar Cycle/1 -> Product/1, Relay/1
  Product/1 -> Scope/2
  From Workspace/1 -> Simulink-PS Converter1/1, Scope/1
  connections:
  Simulink-PS Converter1/RConn1 -- Solar Radiation/RConn1

== system IFACS_Spring2026/House Cooled by Singular Fan, Bang Bang Controller/House Thermal Network/House Thermal Network/Temp Measurements ==
  Celsius to Fahrenheit : simulink_extras/Transformations/Celsius to Fahrenheit
  Celsius to Fahrenheit1 : simulink_extras/Transformations/Celsius to Fahrenheit
  Celsius to Fahrenheit2 : simulink_extras/Transformations/Celsius to Fahrenheit
  PS2S1 : nesl_utility/PS-Simulink Converter  PhysicalDomain=network_engine_domain  SubClassName=ps_output  LeftPortType=input  RightPortType=output  PseudoPeriodic=off  Frequencies=[]  VectorFormat=1-D array  Unit=degC  AffineConversion=on
  PS2S2 : nesl_utility/PS-Simulink Converter  PhysicalDomain=network_engine_domain  SubClassName=ps_output  LeftPortType=input  RightPortType=output  PseudoPeriodic=off  Frequencies=[]  VectorFormat=1-D array  Unit=degC  AffineConversion=on
  PS2S3 : nesl_utility/PS-Simulink Converter  PhysicalDomain=network_engine_domain  SubClassName=ps_output  LeftPortType=input  RightPortType=output  PseudoPeriodic=off  Frequencies=[]  VectorFormat=1-D array  Unit=degC  AffineConversion=on
  TRef2 : fl_lib/Thermal/Thermal Elements/Thermal Reference
  TRef3 : fl_lib/Thermal/Thermal Elements/Thermal Reference
  TRef4 : fl_lib/Thermal/Thermal Elements/Thermal Reference
  Temperature Sensor1 : fl_lib/Thermal/Thermal Sensors/Temperature Sensor  temperature_measure=foundation.enum.MeasurementReference.difference
  Temperature Sensor2 : fl_lib/Thermal/Thermal Sensors/Temperature Sensor  temperature_measure=foundation.enum.MeasurementReference.difference
  Temperature Sensor3 : fl_lib/Thermal/Thermal Sensors/Temperature Sensor  temperature_measure=foundation.enum.MeasurementReference.difference
  Roof Temp : PMIOPort  Side=Left
  Wall Temp : PMIOPort  Port=2  Side=Left
  Window Temp : PMIOPort  Port=3  Side=Left
  Fahrenheit out : Outport
  Fahrenheit out1 : Outport  Port=2
  Fahrenheit out2 : Outport  Port=3
  wires:
  PS2S3/1 -> Celsius to Fahrenheit2/1  "Window"
  PS2S1/1 -> Celsius to Fahrenheit/1  "Roof"
  PS2S2/1 -> Celsius to Fahrenheit1/1  "Wall"
  Celsius to Fahrenheit2/1 -> Fahrenheit out2/1
  Celsius to Fahrenheit1/1 -> Fahrenheit out1/1
  Celsius to Fahrenheit/1 -> Fahrenheit out/1
  connections:
  PS2S2/LConn1 -- Temperature Sensor2/RConn2
  PS2S3/LConn1 -- Temperature Sensor3/RConn2
  TRef2/LConn1 -- Temperature Sensor1/RConn1
  TRef3/LConn1 -- Temperature Sensor2/RConn1
  PS2S1/LConn1 -- Temperature Sensor1/RConn2
  Temperature Sensor2/LConn1 -- Wall Temp/RConn1
  TRef4/LConn1 -- Temperature Sensor3/RConn1
  Temperature Sensor3/LConn1 -- Window Temp/RConn1
  Temperature Sensor1/LConn1 -- Roof Temp/RConn1

== system IFACS_Spring2026/House Cooled by Singular Fan, Proportional Controller/Fan Parameters/Fan Activation/Fan Activation Relays ==
  Tmin : Inport
  Tenv : Inport  Port=2
  Troom : Inport  Port=3
  Cooling Activation : Relay  OnSwitchValue=1  OffSwitchValue=-1
  Product : Product
  Room Temp Min off switch : Relay  OnSwitchValue=2  OffSwitchValue=-2
  Sum1 : Sum  Inputs=-+|  InputSameDT=on  SaturateOnIntegerOverflow=on  OutDataTypeStr=Inherit: Same as first input
  Sum2 : Sum  Inputs=-+|  InputSameDT=on  SaturateOnIntegerOverflow=on  OutDataTypeStr=Inherit: Same as first input
  Fan Activation : Outport
  wires:
  Cooling Activation/1 -> Product/2  "1 if Troom > Tenv else 0"
  Sum2/1 -> Cooling Activation/1  "Terr"
  Tenv/1 -> Sum2/1
  Room Temp Min off switch/1 -> Product/1  "1 if Troom > Tmin else 0"
  Tmin/1 -> Sum1/1
  Troom/1 -> Sum1/2, Sum2/2
  Sum1/1 -> Room Temp Min off switch/1  "Terr"
  Product/1 -> Fan Activation/1

== system IFACS_Spring2026/House Cooled by Singular Fan, Proportional Controller/House Thermal Network/House Thermal Network/Solar Radiation ==
  From Workspace : FromWorkspace  VariableName=time_radiation
  Product : Product
  Relay : Relay  OnSwitchValue=1  OffSwitchValue=0
  Scope : Scope  NumInputPorts=2
      settings: TimeUnits=Metric (based on Time Span)  ActiveDisplayYMinimum=-624.999986167378  ActiveDisplayYMaximum=5624.9998755064025  DataLoggingVariableName=ScopeData2
  Simulink-PS Converter1 : nesl_utility/Simulink-PS Converter  PhysicalDomain=network_engine_domain  SubClassName=ps_input  LeftPortType=input  RightPortType=output  PseudoPeriodic=off  Frequencies=[]  NoiseDistribution=none  NoiseParameters=[]  Unit=1  AffineConversion=off  FilteringAndDerivatives=provide  SimscapeFilterOrder=1  InputFilterTimeConstant=0.001  UdotUserProvided=0
  Solar Cycle : Sin  Amplitude=5000  Frequency=(2*pi)/(24*3600)  SampleTime=0
  Solar Radiation : PMIOPort  Side=Right
  wires:
  Relay/1 -> Product/2
  Solar Cycle/1 -> Product/1, Relay/1
  Product/1 -> Scope/2
  From Workspace/1 -> Simulink-PS Converter1/1, Scope/1
  connections:
  Simulink-PS Converter1/RConn1 -- Solar Radiation/RConn1

== system IFACS_Spring2026/House Cooled by Singular Fan, Proportional Controller/House Thermal Network/House Thermal Network/Temp Measurements ==
  Celsius to Fahrenheit : simulink_extras/Transformations/Celsius to Fahrenheit
  Celsius to Fahrenheit1 : simulink_extras/Transformations/Celsius to Fahrenheit
  Celsius to Fahrenheit2 : simulink_extras/Transformations/Celsius to Fahrenheit
  PS2S1 : nesl_utility/PS-Simulink Converter  PhysicalDomain=network_engine_domain  SubClassName=ps_output  LeftPortType=input  RightPortType=output  PseudoPeriodic=off  Frequencies=[]  VectorFormat=1-D array  Unit=degC  AffineConversion=on
  PS2S2 : nesl_utility/PS-Simulink Converter  PhysicalDomain=network_engine_domain  SubClassName=ps_output  LeftPortType=input  RightPortType=output  PseudoPeriodic=off  Frequencies=[]  VectorFormat=1-D array  Unit=degC  AffineConversion=on
  PS2S3 : nesl_utility/PS-Simulink Converter  PhysicalDomain=network_engine_domain  SubClassName=ps_output  LeftPortType=input  RightPortType=output  PseudoPeriodic=off  Frequencies=[]  VectorFormat=1-D array  Unit=degC  AffineConversion=on
  TRef2 : fl_lib/Thermal/Thermal Elements/Thermal Reference
  TRef3 : fl_lib/Thermal/Thermal Elements/Thermal Reference
  TRef4 : fl_lib/Thermal/Thermal Elements/Thermal Reference
  Temperature Sensor1 : fl_lib/Thermal/Thermal Sensors/Temperature Sensor  temperature_measure=foundation.enum.MeasurementReference.difference
  Temperature Sensor2 : fl_lib/Thermal/Thermal Sensors/Temperature Sensor  temperature_measure=foundation.enum.MeasurementReference.difference
  Temperature Sensor3 : fl_lib/Thermal/Thermal Sensors/Temperature Sensor  temperature_measure=foundation.enum.MeasurementReference.difference
  Roof Temp : PMIOPort  Side=Left
  Wall Temp : PMIOPort  Port=2  Side=Left
  Window Temp : PMIOPort  Port=3  Side=Left
  Fahrenheit out : Outport
  Fahrenheit out1 : Outport  Port=2
  Fahrenheit out2 : Outport  Port=3
  wires:
  PS2S3/1 -> Celsius to Fahrenheit2/1  "Window"
  PS2S1/1 -> Celsius to Fahrenheit/1  "Roof"
  PS2S2/1 -> Celsius to Fahrenheit1/1  "Wall"
  Celsius to Fahrenheit2/1 -> Fahrenheit out2/1
  Celsius to Fahrenheit1/1 -> Fahrenheit out1/1
  Celsius to Fahrenheit/1 -> Fahrenheit out/1
  connections:
  PS2S2/LConn1 -- Temperature Sensor2/RConn2
  PS2S3/LConn1 -- Temperature Sensor3/RConn2
  TRef2/LConn1 -- Temperature Sensor1/RConn1
  TRef3/LConn1 -- Temperature Sensor2/RConn1
  PS2S1/LConn1 -- Temperature Sensor1/RConn2
  Temperature Sensor2/LConn1 -- Wall Temp/RConn1
  TRef4/LConn1 -- Temperature Sensor3/RConn1
  Temperature Sensor3/LConn1 -- Window Temp/RConn1
  Temperature Sensor1/LConn1 -- Roof Temp/RConn1

== system IFACS_Spring2026/House Cooled by simple AC unit/House Thermal Network/House Thermal Network/Solar Radiation ==
  From Workspace : FromWorkspace  VariableName=time_radiation
  Product : Product
  Relay : Relay  OnSwitchValue=1  OffSwitchValue=0
  Scope : Scope  NumInputPorts=2
      settings: TimeUnits=Metric (based on Time Span)  ActiveDisplayYMinimum=-624.999986167378  ActiveDisplayYMaximum=5624.9998755064025  DataLoggingVariableName=ScopeData2
  Simulink-PS Converter1 : nesl_utility/Simulink-PS Converter  PhysicalDomain=network_engine_domain  SubClassName=ps_input  LeftPortType=input  RightPortType=output  PseudoPeriodic=off  Frequencies=[]  NoiseDistribution=none  NoiseParameters=[]  Unit=1  AffineConversion=off  FilteringAndDerivatives=provide  SimscapeFilterOrder=1  InputFilterTimeConstant=0.001  UdotUserProvided=0
  Solar Cycle : Sin  Amplitude=5000  Frequency=(2*pi)/(24*3600)  SampleTime=0
  Solar Radiation : PMIOPort  Side=Right
  wires:
  Relay/1 -> Product/2
  Solar Cycle/1 -> Product/1, Relay/1
  Product/1 -> Scope/2
  From Workspace/1 -> Simulink-PS Converter1/1, Scope/1
  connections:
  Simulink-PS Converter1/RConn1 -- Solar Radiation/RConn1
